simulink model "HITL_DEMO"  (R2021b)
settings: Solver=FixedStepAuto  StartTime=0.0  StopTime=inf  FixedStep=.001  MaxStep=0.01  RelTol=1e-3
libraries: etargetslib x2, instrumentlib x1
settings Model: Creator=kiran  LastModifiedBy=kiran
settings SolverCC: AutoInsertRateTranBlk=on

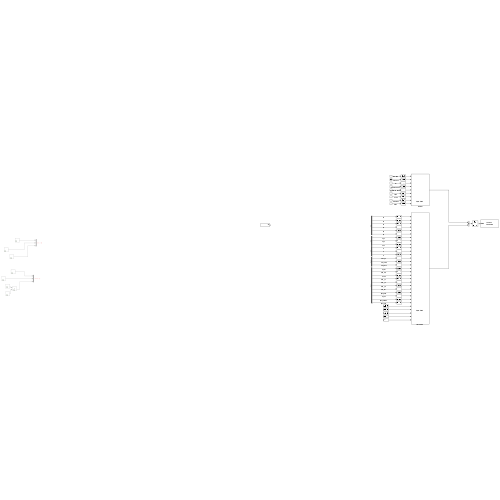
[thumbnail: Simulink's stored preview of the top-level diagram]
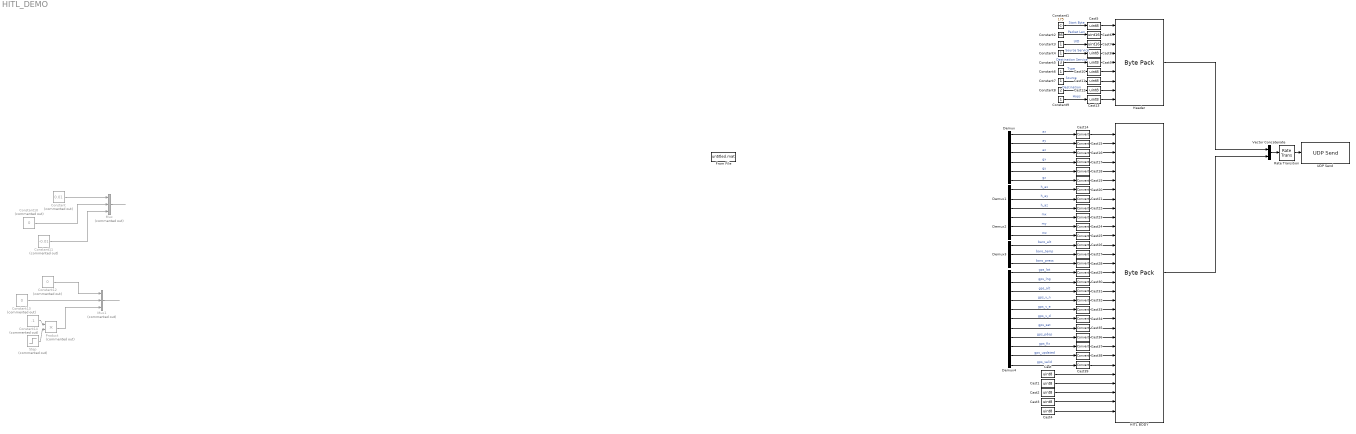
== system HITL_DEMO ==
  Cast{,1..5,8..13} (12 alike) : DataTypeConversion  OutDataTypeStr=uint8
  Cast{14..39} (26 alike) : DataTypeConversion
  Cast6 : DataTypeConversion  OutDataTypeStr=uint16
  Cast7 : DataTypeConversion  OutDataTypeStr=uint16
  Constant : Constant  Commented=on  Value=0.01
  Constant1 : Constant  Value=175
  Constant10 : Constant  Commented=on  Value=0
  Constant11 : Constant  Commented=on  Value=-0.01
  Constant12 : Constant  Commented=on  Value=0
  Constant13 : Constant  Commented=on  Value=0
  Constant14 : Constant  Commented=on  Value=.1
  Constant2 : Constant  Value=95
  Constant{3..4,6..7,9} (5 alike) : Constant
  Constant5 : Constant  Value=3
  Constant8 : Constant  Value=2
  Demux : Demux  Outputs=6
  Demux1 : Demux  Outputs=3
  Demux2 : Demux  Outputs=3
  Demux3 : Demux  Outputs=3
  Demux4 : Demux  Outputs=11
  From File : FromFile  SampleTime=0
  HITL BODY : etargetslib/Byte Pack  datatypes={'single','single','single','single','single','single','single','single','single','single','single','single','single','single','single','single','single','int32','int32','int32','int32','uint8','uint16','uint8','uint8','uint8','uint8','uint8','uint8','uint8','uint8'}  byteAlign=1
  Header : etargetslib/Byte Pack  datatypes={'uint8','uint16','uint16','uint8','uint8','uint8','uint8','uint8','uint8'}  byteAlign=1
  Mux : Mux  Commented=on  Inputs=3
  Mux1 : Mux  Commented=on  Inputs=3
  Product : Product  Commented=on
  Rate Transition : RateTransition  OutPortSampleTime=.01
  Step : Step  Commented=on  Time=10  Before=1  After=0  SampleTime=0
  UDP Send : instrumentlib/UDP Send  Host=127.0.0.1  Port=9090  LocalPort=-1  EnablePortSharing=off  ByteOrder=LittleEndian  OutputDatagramPacketSize=512  EnableBlockingMode=on  LocalAddress=0.0.0.0
  Vector Concatenate : Concatenate
  wires:
  Vector Concatenate/1 -> Rate Transition/1
  Header/1 -> Vector Concatenate/1
  HITL BODY/1 -> Vector Concatenate/2
  Demux/1 -> Cast14/1  "ax"
  Demux/2 -> Cast15/1  "ay"
  Demux/3 -> Cast16/1  "az"
  Demux/4 -> Cast17/1  "gx"
  Demux/6 -> Cast19/1  "gz"
  Demux1/1 -> Cast20/1  "h_ax"
  Demux1/2 -> Cast21/1  "h_ay"
  Demux1/3 -> Cast22/1  "h_az"
  Demux2/1 -> Cast23/1  "mx"
  Demux2/2 -> Cast24/1  "my"
  Demux2/3 -> Cast25/1  "mz"
  Demux3/1 -> Cast26/1  "baro_alt"
  Demux3/2 -> Cast27/1  "baro_temp"
  Demux3/3 -> Cast28/1  "baro_press"
  Demux4/1 -> Cast29/1  "gps_lat"
  Demux4/2 -> Cast30/1  "gps_lng"
  Demux4/3 -> Cast31/1  "gps_alt"
  Demux4/4 -> Cast32/1  "gps_v_n"
  Demux4/5 -> Cast33/1  "gps_v_e"
  Demux4/6 -> Cast34/1  "gps_v_d"
  Demux4/7 -> Cast35/1  "gps_sat"
  Demux4/8 -> Cast36/1  "gps_pdop"
  Demux4/9 -> Cast37/1  "gps_fix"
  Demux4/10 -> Cast38/1  "gps_updated"
  Demux4/11 -> Cast39/1  "gps_valid"
  Demux/5 -> Cast18/1  "gy"
  Constant1/1 -> Cast5/1  "Start Byte"
  Constant2/1 -> Cast6/1  "Packet Len"
  Constant3/1 -> Cast7/1  "UID"
  Constant4/1 -> Cast8/1  "Source Service"
  Constant5/1 -> Cast9/1  "Destination Service"
  Constant6/1 -> Cast10/1  "Type"
  Constant7/1 -> Cast11/1  "Source"
  Constant8/1 -> Cast12/1  "Destination"
  Constant9/1 -> Cast13/1  "Hops"
  Mux/1 -> ?
  Constant/1 -> Mux/1
  Constant10/1 -> Mux/2
  Constant11/1 -> Mux/3
  Product/1 -> Mux1/3
  Constant12/1 -> Mux1/1
  Constant13/1 -> Mux1/2
  Mux1/1 -> ?
  Cast2/1 -> HITL BODY/29
  Cast3/1 -> HITL BODY/30
  Cast4/1 -> HITL BODY/31
  Cast5/1 -> Header/1
  Cast6/1 -> Header/2
  Cast7/1 -> Header/3
  Cast8/1 -> Header/4
  Cast9/1 -> Header/5
  Cast10/1 -> Header/6
  Cast11/1 -> Header/7
  Cast12/1 -> Header/8
  Cast13/1 -> Header/9
  Cast14/1 -> HITL BODY/1
  Cast15/1 -> HITL BODY/2
  Cast16/1 -> HITL BODY/3
  Cast17/1 -> HITL BODY/4
  Cast18/1 -> HITL BODY/5
  Cast19/1 -> HITL BODY/6
  Cast20/1 -> HITL BODY/7
  Cast25/1 -> HITL BODY/12
  Cast23/1 -> HITL BODY/10
  Cast27/1 -> HITL BODY/14
  Cast26/1 -> HITL BODY/13
  Cast22/1 -> HITL BODY/9
  Cast24/1 -> HITL BODY/11
  Cast21/1 -> HITL BODY/8
  Cast39/1 -> HITL BODY/26
  Cast/1 -> HITL BODY/27
  Cast1/1 -> HITL BODY/28
  Cast36/1 -> HITL BODY/23
  Cast38/1 -> HITL BODY/25
  Cast37/1 -> HITL BODY/24
  Cast35/1 -> HITL BODY/22
  Cast33/1 -> HITL BODY/20
  Cast32/1 -> HITL BODY/19
  Cast34/1 -> HITL BODY/21
  Cast31/1 -> HITL BODY/18
  Cast28/1 -> HITL BODY/15
  Cast30/1 -> HITL BODY/17
  Cast29/1 -> HITL BODY/16
  Rate Transition/1 -> UDP Send/1
  Constant14/1 -> Product/1
  Step/1 -> Product/2
